simulink model "aa"  (Simulink 8.2)
settings: Solver=ode15s  StartTime=0.0  StopTime=10.0  RelTol=1e-3
undefined symbols (not defined in the file or in its folder): b, K, R
libraries: fl_lib x10, nesl_utility x5
settings Model: Creator=maen  LastModifiedBy=gyurse

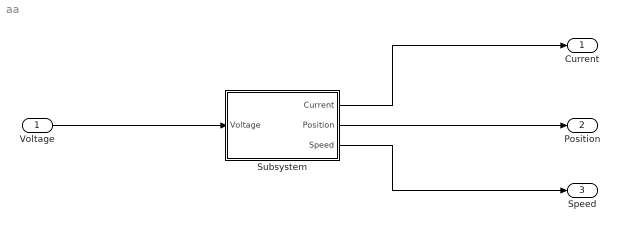
== system aa ==
  Voltage : Inport
  Subsystem : Subsystem
  Current : Outport
  Position : Outport  Port=2
  Speed : Outport  Port=3
  wires:
  Subsystem/1(Current) -> Current/1
  Voltage/1 -> Subsystem/1(Voltage)
  Subsystem/2(Position) -> Position/1
  Subsystem/3(Speed) -> Speed/1

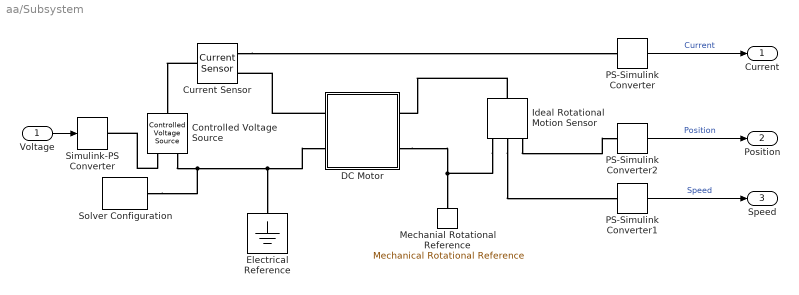
== system aa/Subsystem ==
  Voltage : Inport
  Controlled Voltage Source : fl_lib/Electrical/Electrical Sources/Controlled Voltage Source  i_Log=off  v_Log=off  LocalVarNames=|i|v  LocalVarDescs=|i|v  LocalVarLogging=[0 0]
  Current Sensor : fl_lib/Electrical/Electrical Sensors/Current Sensor  i1_Log=off  v1_Log=off  LocalVarNames=|i1|v1  LocalVarDescs=|i1|v1  LocalVarLogging=[0 0]
  DC Motor : Subsystem
  Electrical Reference : fl_lib/Electrical/Electrical Elements/Electrical Reference  i_Log=off  LocalVarNames=|i  LocalVarDescs=|i  LocalVarLogging=0
  Ideal Rotational Motion Sensor : fl_lib/Mechanical/Mechanical Sensors/Ideal Rotational Motion Sensor  offset=0 rad  w_Log=off  t_Log=off  phi_Log=off  LocalVarNames=|w|t|phi  LocalVarDescs=|w|t|phi  LocalVarLogging=[0 0 0]
  Mechanial Rotational Reference : fl_lib/Mechanical/Rotational Elements/Mechanical Rotational Reference  t_Log=off  LocalVarNames=|t  LocalVarDescs=|t  LocalVarLogging=0
  PS-Simulink Converter : nesl_utility/PS-Simulink Converter  PhysicalDomain=network_engine_domain  SubClassName=ps_output  LeftPortType=input  RightPortType=output  PseudoPeriodic=off  Frequencies=[]  Unit=1  AffineConversion=off
  PS-Simulink Converter1 : nesl_utility/PS-Simulink Converter  PhysicalDomain=network_engine_domain  SubClassName=ps_output  LeftPortType=input  RightPortType=output  PseudoPeriodic=off  Frequencies=[]  Unit=1  AffineConversion=off
  PS-Simulink Converter2 : nesl_utility/PS-Simulink Converter  PhysicalDomain=network_engine_domain  SubClassName=ps_output  LeftPortType=input  RightPortType=output  PseudoPeriodic=off  Frequencies=[]  Unit=rad  AffineConversion=off
  Simulink-PS Converter : nesl_utility/Simulink-PS Converter  PhysicalDomain=network_engine_domain  SubClassName=ps_input  LeftPortType=input  RightPortType=output  PseudoPeriodic=off  Frequencies=[]  NoiseDistribution=none  NoiseParameters=[]  Unit=V  AffineConversion=off  InputFiltering=off  SimscapeFilterOrder=1  InputFilterTimeConstant=.001  UdotUserProvided=0
  Solver Configuration : nesl_utility/Solver Configuration  PhysicalDomain=network_engine_domain  SubClassName=solver  LeftPortType=input  RightPortType=generic  Accelerate=off  Tones=[]  Harmonics=[]  SimulateNoise=off  Profile=off  UseLocalSampling=off  EnableSwitchedLinearOptims=on  FrequencyDomain=off  UseCCode=off  RelTol=0.001  AbsTol=1e-06  MinStep=1e-09  ToWorkspace=off  DoDC=off  ResidualTolerance=1e-9  UseLocalSolver=off  LocalSolverChoice=NE_BACKWARD_EULER_ADVANCER  LocalSolverSampleTime=.001  DoFixedCost=off  MaxNonlinIter=3  MaxModeIter=2  LinearAlgebra=Sparse  DelaysMemoryBudget=1024
  Current : Outport
  Position : Outport  Port=2
  Speed : Outport  Port=3
  wires:
  PS-Simulink Converter/1 -> Current/1  "Current"
  PS-Simulink Converter1/1 -> Speed/1  "Speed"
  Voltage/1 -> Simulink-PS Converter/1
  PS-Simulink Converter2/1 -> Position/1  "Position"
  connections:
  Current Sensor/LConn1 -- Controlled Voltage Source/LConn1
  Controlled Voltage Source/RConn1 -- Simulink-PS Converter/RConn1
  Controlled Voltage Source/RConn2 -- DC Motor/LConn2 -- Electrical Reference/LConn1 -- Solver Configuration/RConn1
  Current Sensor/RConn1 -- PS-Simulink Converter/LConn1
  DC Motor/LConn1 -- Current Sensor/RConn2
  Ideal Rotational Motion Sensor/LConn1 -- DC Motor/RConn1
  DC Motor/RConn2 -- Ideal Rotational Motion Sensor/RConn1 -- Mechanial Rotational Reference/LConn1
  Ideal Rotational Motion Sensor/RConn2 -- PS-Simulink Converter1/LConn1
  Ideal Rotational Motion Sensor/RConn3 -- PS-Simulink Converter2/LConn1

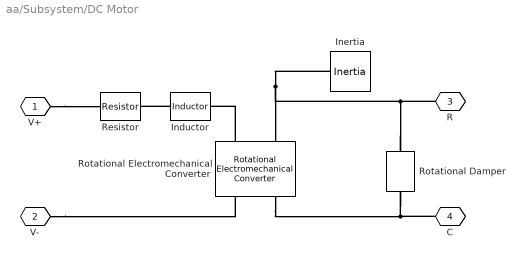
== system aa/Subsystem/DC Motor ==
  Inductor : fl_lib/Electrical/Electrical Elements/Inductor  l=L H  i0=0 A  r=0 Ohm  g=1e-9 1/Ohm  i_Log=off  v_Log=off  i_L_Log=off  LocalVarNames=|i|v|i_L  LocalVarDescs=|i|v|Internal variable for current through inductor term  LocalVarLogging=[0 0 0]
  Inertia : fl_lib/Mechanical/Rotational Elements/Inertia  inertia=J kg*m^2  initial_velocity=0 rad/s  t_Log=off  LocalVarNames=|t  LocalVarDescs=|t  LocalVarLogging=0
  Resistor : fl_lib/Electrical/Electrical Elements/Resistor  R=R Ohm  i_Log=off  v_Log=off  LocalVarNames=|i|v  LocalVarDescs=|i|v  LocalVarLogging=[0 0]
  Rotational Electromechanical Converter : fl_lib/Electrical/Electrical Elements/Rotational Electromechanical Converter  K=K V/(rad/s)  i_Log=off  v_Log=off  t_Log=off  w_Log=off  LocalVarNames=|i|v|t|w  LocalVarDescs=|i|v|t|w  LocalVarLogging=[0 0 0 0]
  Rotational Damper : fl_lib/Mechanical/Rotational Elements/Rotational Damper  D=b N*m/(rad/s)  t_Log=off  w_Log=off  LocalVarNames=|t|w  LocalVarDescs=|t|w  LocalVarLogging=[0 0]
  V+ : PMIOPort  Tag=PMCPort  Port=1  Side=Left
  V- : PMIOPort  Tag=PMCPort  Port=2  Side=Left
  R : PMIOPort  Tag=PMCPort  Port=3  Side=Right
  C : PMIOPort  Tag=PMCPort  Port=4  Side=Right
  connections:
  Inductor/LConn1 -- Resistor/RConn1
  Rotational Electromechanical Converter/LConn1 -- Inductor/RConn1
  Rotational Damper/LConn1 -- R/RConn1 -- Inertia/LConn1 -- Rotational Electromechanical Converter/LConn2
  V+/RConn1 -- Resistor/LConn1
  V-/RConn1 -- Rotational Electromechanical Converter/RConn1
  Rotational Damper/RConn1 -- C/RConn1 -- Rotational Electromechanical Converter/RConn2
